simulink model "CxTh_Suff_Neurosci_2004"  (Simulink 6.2)
settings: Solver=ode5  SolverMode=SingleTasking  StartTime=0.0  StopTime=30  FixedStep=0.001  MaxStep=0.01  RelTol=1e-3
libraries: simulink x18
settings Model: LastModifiedBy=Piotr Suffczynski  ExtModeAutoUpdateStatusClock=off
settings SolverCC: InitialStep=0.001
settings DataIOCC: SaveOutput=off  SaveTime=off  SignalLoggingName=sigsOut
settings OptimizationCC: BooleanDataType=off
settings DebuggingCC: CheckMatrixSingularityMsg=warning
settings HardwareCC: TargetUnknown=on
settings GRTTargetCC: ModelReferenceCompliant=off  MatFileLogging=off

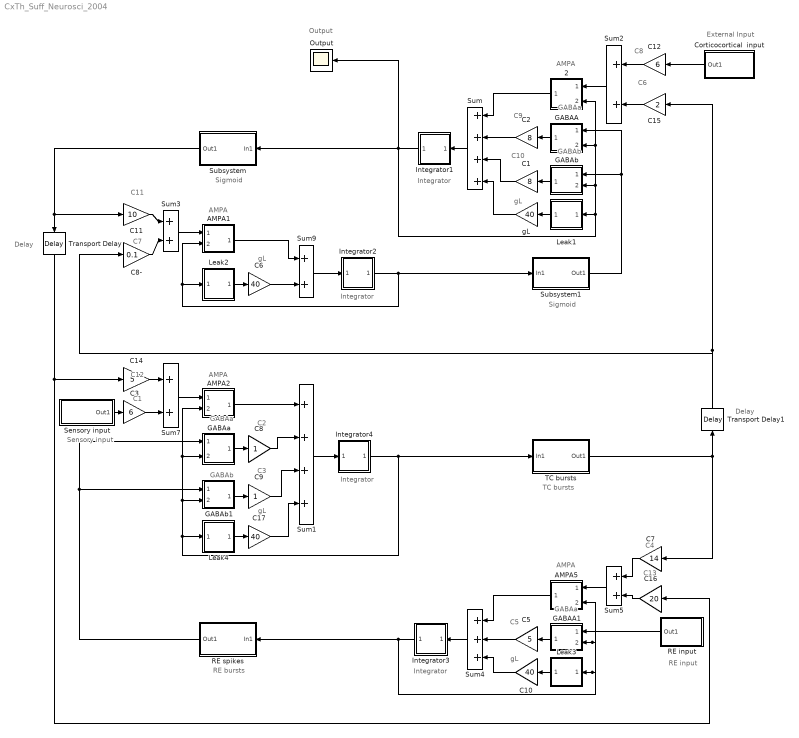
== system CxTh_Suff_Neurosci_2004 ==
  note: Integrator
  note: GABAa
  note: GABAb
  note: AMPA
  note: Sigmoid
  note: AMPA
  note: GABAb
  note: GABAa
  note: AMPA
  note: GABAa
  note: AMPA
  note: External Input
  note: Delay
  note: Delay
  note: Sensory input
  note: RE input
  note: Integrator
  note: Integrator
  note: Integrator
  note: TC bursts
  note: RE bursts
  note: C1
  note: C2
  note: C3
  note: gL
  note: gL
  note: C4
  note: C5
  note: gL
  note: C6
  note: C7
  note: C8
  note: C9
  note: C10
  note: gL
  note: C11
  note: C12
  note: C13
  note: Sigmoid
  note: Output
  2 : Subsystem  Orientation=left
      mask Display: plot([0 5 10 15 20 30 40 60 80 100 150 350], [0  0.3 0.8 1 0.75 0.42 0.22 0.1 0.03 0.01 0 0])
  AMPA1 : Subsystem
      mask Display: plot([0 5 10 15 20 30 40 60 80 100 150 350], [0  0.3 0.8 1 0.75 0.42 0.22 0.1 0.03 0.01 0 0])
  AMPA2 : Subsystem
      mask Display: plot([0 5 10 15 20 30 40 60 80 100 150 350], [0  0.3 0.8 1 0.75 0.42 0.22 0.1 0.03 0.01 0 0])
  AMPA5 : Subsystem  Orientation=left
      mask Display: plot([0 5 10 15 20 30 40 60 80 100 150 350], [0  0.3 0.8 1 0.75 0.42 0.22 0.1 0.03 0.01 0 0])
  C1 : Gain  Orientation=left  Gain=8  SaturateOnIntegerOverflow=on
  C10 : Gain  Orientation=left  Gain=40  SaturateOnIntegerOverflow=on
  C11 : Gain  Gain=10  SaturateOnIntegerOverflow=on
  C12 : Gain  Orientation=left  Gain=6  SaturateOnIntegerOverflow=on
  C14 : Gain  Gain=5  SaturateOnIntegerOverflow=on
  C15 : Gain  Orientation=left  Gain=2  SaturateOnIntegerOverflow=on
  C16 : Gain  Orientation=left  Gain=20  SaturateOnIntegerOverflow=on
  C17 : Gain  Gain=40  SaturateOnIntegerOverflow=on
  C2 : Gain  Orientation=left  Gain=8  SaturateOnIntegerOverflow=on
  C3 : Gain  Gain=6  SaturateOnIntegerOverflow=on
  C5 : Gain  Orientation=left  Gain=5  SaturateOnIntegerOverflow=on
  C6 : Gain  Gain=40  SaturateOnIntegerOverflow=on
  C7 : Gain  Orientation=left  Gain=14  SaturateOnIntegerOverflow=on
  C8 : Gain  SaturateOnIntegerOverflow=on
  C8- : Gain  Gain=0.1
  C9 : Gain  SaturateOnIntegerOverflow=on
  Corticocortical  input : Subsystem  Orientation=left
      mask Display: plot([1 2 3 4 5 6 7 8 9 10 11 12],[0 3 -2 5 1 -2 6 -4 -1 2 -1 0])
  GABAA : Subsystem  Orientation=left
      mask Display: plot([10 15 20 30 40 60 80 100 150 350], [0  0.5 1 0.75 0.5 0.3 0.2 0.1 0.01 0 ])
  GABAA1 : Subsystem  Orientation=left
      mask Display: plot([10 15 20 30 40 60 80 100 150 350], [0  0.5 1 0.75 0.5 0.3 0.2 0.1 0.01 0 ])
  GABAa : Subsystem
      mask Display: plot([10 15 20 30 40 60 80 100 150 350], [0  0.5 1 0.75 0.5 0.3 0.2 0.1 0.01 0 ])
  GABAb : Subsystem  Orientation=left
      mask Display:
      | plot([0 10 20 30 40 50 60 70 80 90 100 125 150 200 250 300],
      | [0 3 7 8  7.5 6.5 5.5 4.5 3.5 2.8 2.2 1.2 0.6 0.2 0.1 0])
  GABAb1 : Subsystem
      mask Display:
      | plot([0 10 20 30 40 50 60 70 80 90 100 125 150 200 250 300],
      | [0 3 7 8  7.5 6.5 5.5 4.5 3.5 2.8 2.2 1.2 0.6 0.2 0.1 0])
  Integrator1 : Subsystem  Orientation=left
      mask Display:
      | plot([ 1 2 3 4 5 6 7 8 9 10 ] - 2,
      |  [0 0 0.5  2  4 6 8  9.5 10 10], -4, 0, 15, 10 )
      | disp('    dt')
  Integrator2 : Subsystem
      mask Display:
      | plot([ 1 2 3 4 5 6 7 8 9 10 ] - 2,
      |  [0 0 0.5  2  4 6 8  9.5 10 10], -4, 0, 15, 10 )
      | disp('    dt')
  Integrator3 : Subsystem  Orientation=left
      mask Display:
      | plot([ 1 2 3 4 5 6 7 8 9 10 ] - 2,
      |  [0 0 0.5  2  4 6 8  9.5 10 10], -4, 0, 15, 10 )
      | disp('    dt')
  Integrator4 : Subsystem
      mask Display:
      | plot([ 1 2 3 4 5 6 7 8 9 10 ] - 2,
      |  [0 0 0.5  2  4 6 8  9.5 10 10], -4, 0, 15, 10 )
      | disp('    dt')
  Leak1 : Subsystem  Orientation=left
      mask Display: disp('Leak')
  Leak2 : Subsystem
      mask Display: disp('Leak')
  Leak3 : Subsystem  Orientation=left
      mask Display: disp('Leak')
  Leak4 : Subsystem
      mask Display: disp('Leak')
  Output : Scope
      settings: TickLabels=on  TimeRange=5  YMin=-1.5  YMax=2  SaveName=V_Cx  DataFormat=Array  MaxDataPoints=100000
  RE input : Subsystem  Orientation=left
      mask Display: plot([0 0 0 20 30 40],[ 0 1 0.3 0.3 0.3 0.3])
  RE spikes : Subsystem  Orientation=left
      mask Display:
      | plot([0 10 20 30 40 50 60 70 80 90 100 110 120 130 140 150 160],
      | [0 0 1 1.9  3.5 5 5.25 5.5 4.5 3.8 3.3 2.2 1.2 0.6 0.2 0.1 0])
      | 
      | plot([50 50], [5 20],  [54 54], [5.1 20], [58 58], [5.2 20], [62 62], [5.3 20], [66 66], [5.4 20],   [70 70], [5.5 20] )
  Sensory input : Subsystem
      mask Display: plot([1 2 3 4 5 6 7 8 9 10 11 12],[0 3 -7 3 -1 2 5 -6 4 2 -4 0])
  Subsystem : Subsystem  Orientation=left
      mask Display:
      | plot(-[0 1 2 3 4 5 6 7 8 9 10 11],
      |  [0 0 0 0.5  2  4 6 8  9.5 10 10 10], 0.1, 0, -10.1, 10 )
  Subsystem1 : Subsystem
      mask Display:
      | plot([0 1 2 3 4 5 6 7 8 9 10 11],
      |  [0 0 0 0.5  2  4 6 8  9.5 10 10 10], -0.1, 0, 10.1, 10 )
  Sum : Sum  Orientation=left  Inputs=++++  SaturateOnIntegerOverflow=on  InputSameDT=on
  Sum1 : Sum  Inputs=4  SaturateOnIntegerOverflow=on  InputSameDT=on
  Sum2 : Sum  Orientation=left  SaturateOnIntegerOverflow=on  InputSameDT=on
  Sum3 : Sum  SaturateOnIntegerOverflow=on  InputSameDT=on
  Sum4 : Sum  Orientation=left  Inputs=+++  SaturateOnIntegerOverflow=on  InputSameDT=on
  Sum5 : Sum  Orientation=left  SaturateOnIntegerOverflow=on  InputSameDT=on
  Sum7 : Sum  SaturateOnIntegerOverflow=on  InputSameDT=on
  Sum9 : Sum  SaturateOnIntegerOverflow=on  InputSameDT=on
  TC bursts : Subsystem
      mask Display:
      | plot([0 10 20 30 40 50 60 70 80 90 100 110 120 130 140 150 160],
      | [0 0 1 1.9  3.5 5 5.25 5.5 4.5 3.8 3.3 2.2 1.2 0.6 0.2 0.1 0])
      | 
      | plot([50 50], [5 20],  [54 54], [5.1 20], [58 58], [5.2 20], [62 62], [5.3 20], [66 66], [5.4 20],   [70 70], [5.5 20] )
  Transport Delay : TransportDelay  Orientation=down  DelayTime=0.008
  Transport Delay1 : TransportDelay  Orientation=up  DelayTime=0.008
  gL : Gain  Orientation=left  Gain=40  SaturateOnIntegerOverflow=on
  wires:
  C8-/1 -> Sum3/2
  C11/1 -> Sum3/1
  Sum3/1 -> AMPA1/1(In1)
  GABAA/1(Out1) -> C2/1
  GABAb/1(Out1) -> C1/1
  Sum/1 -> Integrator1/1(In1)
  Integrator2/1(Out1) -> AMPA1/2(In2), Leak2/1(In2), Subsystem1/1(In1)
  Subsystem1/1(Out1) -> GABAA/1(In1), GABAb/1(In1)
  Sum2/1 -> 2/1(In1)
  C15/1 -> Sum2/2
  RE spikes/1(Out1) -> GABAa/1(In1), GABAb1/1(In1)
  RE input/1(Out1) -> GABAA1/1(In1)
  Sum1/1 -> Integrator4/1(In1)
  TC bursts/1(Out1) -> Transport Delay1/1, C7/1
  GABAb1/1(Out1) -> C9/1
  GABAa/1(Out1) -> C8/1
  AMPA5/1(Out1) -> Sum4/1
  Sum4/1 -> Integrator3/1(In1)
  C7/1 -> Sum5/1
  AMPA2/1(Out1) -> Sum1/1
  Sum7/1 -> AMPA2/1(In1)
  C14/1 -> Sum7/1
  Leak4/1(Out1) -> C17/1
  C17/1 -> Sum1/4
  Transport Delay/1 -> C16/1, C14/1
  Transport Delay1/1 -> C15/1, C8-/1
  C2/1 -> Sum/2
  C1/1 -> Sum/3
  Subsystem/1(Out1) -> Transport Delay/1, C11/1
  C8/1 -> Sum1/2
  C9/1 -> Sum1/3
  Leak1/1(Out1) -> gL/1
  gL/1 -> Sum/4
  Leak2/1(Out1) -> C6/1
  C6/1 -> Sum9/2
  Sum9/1 -> Integrator2/1(In1)
  Leak3/1(Out1) -> C10/1
  C10/1 -> Sum4/3
  C16/1 -> Sum5/2
  Integrator4/1(Out1) -> GABAa/2(In2), AMPA2/2(In2), GABAb1/2(In2), Leak4/1(In2), TC bursts/1(In1)
  Integrator3/1(Out1) -> RE spikes/1(In1), AMPA5/2(In2), GABAA1/2(In2), Leak3/1(In2)
  Sum5/1 -> AMPA5/1(In1)
  2/1(Out1) -> Sum/1
  AMPA1/1(Out1) -> Sum9/1
  C5/1 -> Sum4/2
  GABAA1/1(Out1) -> C5/1
  Integrator1/1(Out1) -> Subsystem/1(In1), Leak1/1(In2), GABAb/2(In2), 2/2(In2), GABAA/2(In2), Output/1
  C3/1 -> Sum7/2
  Sensory input/1(Out1) -> C3/1
  Corticocortical  input/1(Out1) -> C12/1
  C12/1 -> Sum2/1

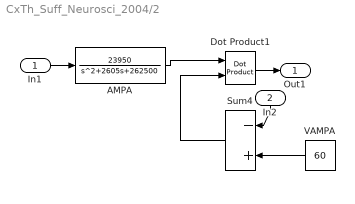
== system CxTh_Suff_Neurosci_2004/2 ==
  In1 : Inport  Port=1  LatchInput=off
  In2 : Inport  Orientation=down  Port=2  LatchInput=off
  AMPA : TransferFcn  Numerator=[23950]  Denominator="[1  2605 262500]"
  Dot Product1 : simulink/Math Operations/Dot Product  InputSameDT=on  OutDataType=sfix(16)  OutScaling=2^-10  DoSatur=off
  Sum4 : Sum  Orientation=left  Inputs=-+  SaturateOnIntegerOverflow=on  InputSameDT=on
  VAMPA : Constant  Orientation=left  Value=60
  Out1 : Outport
  wires:
  Dot Product1/1 -> Out1/1
  In1/1 -> AMPA/1
  In2/1 -> Sum4/1
  Sum4/1 -> Dot Product1/2
  VAMPA/1 -> Sum4/2
  AMPA/1 -> Dot Product1/1

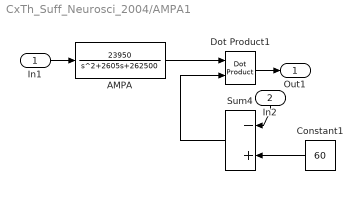
== system CxTh_Suff_Neurosci_2004/AMPA1 ==
  In1 : Inport  Port=1  LatchInput=off
  In2 : Inport  Orientation=down  Port=2  LatchInput=off
  AMPA : TransferFcn  Numerator=[23950]  Denominator="[1  2605 262500]"
  Constant1 : Constant  Orientation=left  Value=60
  Dot Product1 : simulink/Math Operations/Dot Product  InputSameDT=on  OutDataType=sfix(16)  OutScaling=2^-10  DoSatur=off
  Sum4 : Sum  Orientation=left  Inputs=-+  SaturateOnIntegerOverflow=on  InputSameDT=on
  Out1 : Outport
  wires:
  AMPA/1 -> Dot Product1/1
  Constant1/1 -> Sum4/2
  Sum4/1 -> Dot Product1/2
  In2/1 -> Sum4/1
  In1/1 -> AMPA/1
  Dot Product1/1 -> Out1/1

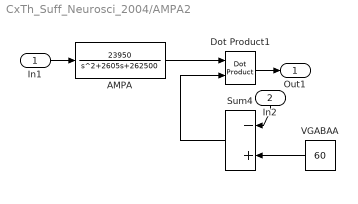
== system CxTh_Suff_Neurosci_2004/AMPA2 ==
  In1 : Inport  Port=1  LatchInput=off
  In2 : Inport  Orientation=down  Port=2  LatchInput=off
  AMPA : TransferFcn  Numerator=[23950]  Denominator="[1  2605 262500]"
  Dot Product1 : simulink/Math Operations/Dot Product  InputSameDT=on  OutDataType=sfix(16)  OutScaling=2^-10  DoSatur=off
  Sum4 : Sum  Orientation=left  Inputs=-+  SaturateOnIntegerOverflow=on  InputSameDT=on
  VGABAA : Constant  Orientation=left  Value=60
  Out1 : Outport
  wires:
  Dot Product1/1 -> Out1/1
  In1/1 -> AMPA/1
  In2/1 -> Sum4/1
  Sum4/1 -> Dot Product1/2
  VGABAA/1 -> Sum4/2
  AMPA/1 -> Dot Product1/1

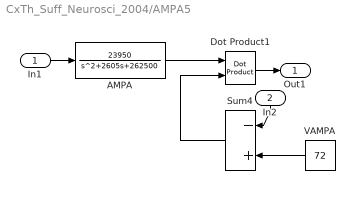
== system CxTh_Suff_Neurosci_2004/AMPA5 ==
  In1 : Inport  Port=1  LatchInput=off
  In2 : Inport  Orientation=down  Port=2  LatchInput=off
  AMPA : TransferFcn  Numerator=[23950]  Denominator="[1  2605 262500]"
  Dot Product1 : simulink/Math Operations/Dot Product  InputSameDT=on  OutDataType=sfix(16)  OutScaling=2^-10  DoSatur=off
  Sum4 : Sum  Orientation=left  Inputs=-+  SaturateOnIntegerOverflow=on  InputSameDT=on
  VAMPA : Constant  Orientation=left  Value=72
  Out1 : Outport
  wires:
  AMPA/1 -> Dot Product1/1
  VAMPA/1 -> Sum4/2
  Sum4/1 -> Dot Product1/2
  In2/1 -> Sum4/1
  In1/1 -> AMPA/1
  Dot Product1/1 -> Out1/1

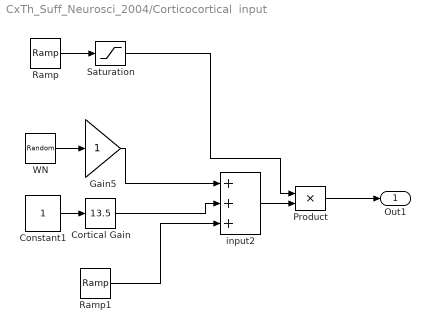
== system CxTh_Suff_Neurosci_2004/Corticocortical  input ==
  Constant1 : Constant
  Cortical Gain : simulink/Math Operations/Slider Gain  low=0  gain=13.5  high=200
  Gain5 : Gain  SaturateOnIntegerOverflow=on
  Product : Product  SaturateOnIntegerOverflow=on  InputSameDT=on
  Ramp : simulink/Sources/Ramp  slope=0.2  start=0  X0=0
  Ramp1 : simulink/Sources/Ramp  slope=0  start=0  X0=0
  Saturation : Saturate  UpperLimit=1  LowerLimit=0
  WN : RandomNumber  SampleTime=0.001
  input2 : Sum  Inputs=+++  SaturateOnIntegerOverflow=on  InputSameDT=on
  Out1 : Outport  InitialOutput=0
  wires:
  Cortical Gain/1 -> input2/2
  WN/1 -> Gain5/1
  Gain5/1 -> input2/1
  Constant1/1 -> Cortical Gain/1
  Saturation/1 -> Product/1
  Ramp/1 -> Saturation/1
  input2/1 -> Product/2
  Product/1 -> Out1/1
  Ramp1/1 -> input2/3

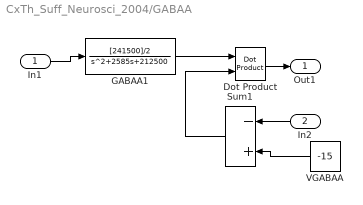
== system CxTh_Suff_Neurosci_2004/GABAA ==
  In1 : Inport  Port=1  LatchInput=off
  In2 : Inport  Orientation=left  Port=2  LatchInput=off
  Dot Product : simulink/Math Operations/Dot Product  InputSameDT=on  OutDataType=sfix(16)  OutScaling=2^-10  DoSatur=off
  GABAA1 : TransferFcn  Numerator=[241500]/2  Denominator="[1  2585 212500]"
  Sum1 : Sum  Orientation=left  Inputs=-+  SaturateOnIntegerOverflow=on  InputSameDT=on
  VGABAA : Constant  Orientation=left  Value=-15
  Out1 : Outport
  wires:
  GABAA1/1 -> Dot Product/1
  VGABAA/1 -> Sum1/2
  Sum1/1 -> Dot Product/2
  In1/1 -> GABAA1/1
  In2/1 -> Sum1/1
  Dot Product/1 -> Out1/1

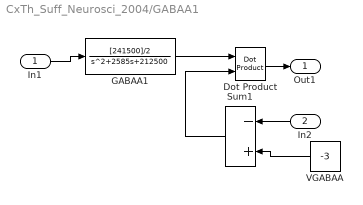
== system CxTh_Suff_Neurosci_2004/GABAA1 ==
  In1 : Inport  Port=1  LatchInput=off
  In2 : Inport  Orientation=left  Port=2  LatchInput=off
  Dot Product : simulink/Math Operations/Dot Product  InputSameDT=on  OutDataType=sfix(16)  OutScaling=2^-10  DoSatur=off
  GABAA1 : TransferFcn  Numerator=[241500]/2  Denominator="[1  2585 212500]"
  Sum1 : Sum  Orientation=left  Inputs=-+  SaturateOnIntegerOverflow=on  InputSameDT=on
  VGABAA : Constant  Orientation=left  Value=-3
  Out1 : Outport
  wires:
  Dot Product/1 -> Out1/1
  In2/1 -> Sum1/1
  In1/1 -> GABAA1/1
  Sum1/1 -> Dot Product/2
  VGABAA/1 -> Sum1/2
  GABAA1/1 -> Dot Product/1

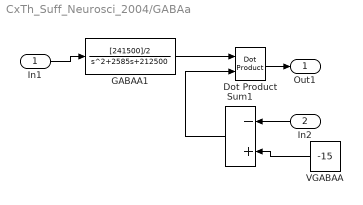
== system CxTh_Suff_Neurosci_2004/GABAa ==
  In1 : Inport  Port=1  LatchInput=off
  In2 : Inport  Orientation=left  Port=2  LatchInput=off
  Dot Product : simulink/Math Operations/Dot Product  InputSameDT=on  OutDataType=sfix(16)  OutScaling=2^-10  DoSatur=off
  GABAA1 : TransferFcn  Numerator=[241500]/2  Denominator="[1  2585 212500]"
  Sum1 : Sum  Orientation=left  Inputs=-+  SaturateOnIntegerOverflow=on  InputSameDT=on
  VGABAA : Constant  Orientation=left  Value=-15
  Out1 : Outport
  wires:
  GABAA1/1 -> Dot Product/1
  VGABAA/1 -> Sum1/2
  Sum1/1 -> Dot Product/2
  In1/1 -> GABAA1/1
  In2/1 -> Sum1/1
  Dot Product/1 -> Out1/1

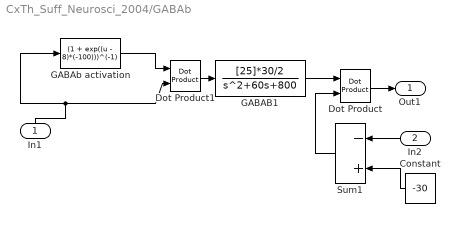
== system CxTh_Suff_Neurosci_2004/GABAb ==
  In1 : Inport  Orientation=up  Port=1  LatchInput=off
  In2 : Inport  Orientation=left  Port=2  LatchInput=off
  Constant : Constant  Orientation=left  Value=-30
  Dot Product : simulink/Math Operations/Dot Product  InputSameDT=on  OutDataType=sfix(16)  OutScaling=2^-10  DoSatur=off
  Dot Product1 : simulink/Math Operations/Dot Product  InputSameDT=on  OutDataType=sfix(16)  OutScaling=2^-10  DoSatur=off
  GABAB1 : TransferFcn  Numerator=[25]*30/2  Denominator="[1  60 800]"
  GABAb activation : Fcn  Expr=(1 + exp((u - 8)*(-100)))^(-1)
  Sum1 : Sum  Orientation=left  Inputs=-+  SaturateOnIntegerOverflow=on  InputSameDT=on
  Out1 : Outport
  wires:
  GABAB1/1 -> Dot Product/1
  Constant/1 -> Sum1/2
  Sum1/1 -> Dot Product/2
  Dot Product1/1 -> GABAB1/1
  In1/1 -> Dot Product1/2, GABAb activation/1
  In2/1 -> Sum1/1
  Dot Product/1 -> Out1/1
  GABAb activation/1 -> Dot Product1/1

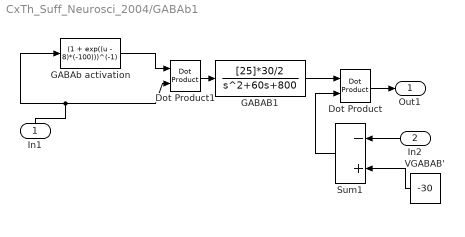
== system CxTh_Suff_Neurosci_2004/GABAb1 ==
  In1 : Inport  Orientation=up  Port=1  LatchInput=off
  In2 : Inport  Orientation=left  Port=2  LatchInput=off
  Dot Product : simulink/Math Operations/Dot Product  InputSameDT=on  OutDataType=sfix(16)  OutScaling=2^-10  DoSatur=off
  Dot Product1 : simulink/Math Operations/Dot Product  InputSameDT=on  OutDataType=sfix(16)  OutScaling=2^-10  DoSatur=off
  GABAB1 : TransferFcn  Numerator=[25]*30/2  Denominator="[1  60 800]"
  GABAb activation : Fcn  Expr=(1 + exp((u - 8)*(-100)))^(-1)
  Sum1 : Sum  Orientation=left  Inputs=-+  SaturateOnIntegerOverflow=on  InputSameDT=on
  VGABAB' : Constant  Orientation=left  Value=-30
  Out1 : Outport
  wires:
  GABAb activation/1 -> Dot Product1/1
  Dot Product/1 -> Out1/1
  In2/1 -> Sum1/1
  In1/1 -> GABAb activation/1, Dot Product1/2
  Dot Product1/1 -> GABAB1/1
  Sum1/1 -> Dot Product/2
  VGABAB'/1 -> Sum1/2
  GABAB1/1 -> Dot Product/1

== system CxTh_Suff_Neurosci_2004/Integrator1 ==
  In1 : Inport  Port=1  LatchInput=off
  Integrator2 : Integrator
  Out1 : Outport
  wires:
  In1/1 -> Integrator2/1
  Integrator2/1 -> Out1/1

== system CxTh_Suff_Neurosci_2004/Integrator2 ==
  In1 : Inport  Port=1  LatchInput=off
  Integrator2 : Integrator
  Out1 : Outport
  wires:
  Integrator2/1 -> Out1/1
  In1/1 -> Integrator2/1

== system CxTh_Suff_Neurosci_2004/Integrator3 ==
  In1 : Inport  Port=1  LatchInput=off
  Integrator2 : Integrator
  Out1 : Outport
  wires:
  Integrator2/1 -> Out1/1
  In1/1 -> Integrator2/1

== system CxTh_Suff_Neurosci_2004/Integrator4 ==
  In1 : Inport  Port=1  LatchInput=off
  Integrator2 : Integrator
  Out1 : Outport
  wires:
  In1/1 -> Integrator2/1
  Integrator2/1 -> Out1/1

== system CxTh_Suff_Neurosci_2004/Leak1 ==
  In2 : Inport  Orientation=left  Port=1  LatchInput=off
  Sum1 : Sum  Orientation=left  Inputs=-+  SaturateOnIntegerOverflow=on  InputSameDT=on
  Vleak : Constant  Orientation=left  Value=0
  Out1 : Outport
  wires:
  Vleak/1 -> Sum1/2
  In2/1 -> Sum1/1
  Sum1/1 -> Out1/1

== system CxTh_Suff_Neurosci_2004/Leak2 ==
  In2 : Inport  Orientation=left  Port=1  LatchInput=off
  Sum1 : Sum  Orientation=left  Inputs=-+  SaturateOnIntegerOverflow=on  InputSameDT=on
  Vleak : Constant  Orientation=left  Value=0
  Out1 : Outport
  wires:
  Sum1/1 -> Out1/1
  In2/1 -> Sum1/1
  Vleak/1 -> Sum1/2

== system CxTh_Suff_Neurosci_2004/Leak3 ==
  In2 : Inport  Orientation=left  Port=1  LatchInput=off
  Sum1 : Sum  Orientation=left  Inputs=-+  SaturateOnIntegerOverflow=on  InputSameDT=on
  Vleak : Constant  Orientation=left  Value=0
  Out1 : Outport
  wires:
  Vleak/1 -> Sum1/2
  In2/1 -> Sum1/1
  Sum1/1 -> Out1/1

== system CxTh_Suff_Neurosci_2004/Leak4 ==
  In2 : Inport  Orientation=left  Port=1  LatchInput=off
  Sum1 : Sum  Orientation=left  Inputs=-+  SaturateOnIntegerOverflow=on  InputSameDT=on
  Vleak : Constant  Orientation=left  Value=0
  Out1 : Outport
  wires:
  Vleak/1 -> Sum1/2
  In2/1 -> Sum1/1
  Sum1/1 -> Out1/1

== system CxTh_Suff_Neurosci_2004/RE input ==
  Constant2 : Constant  Orientation=left  Value=12
  Out1 : Outport  Orientation=left
  wires:
  Constant2/1 -> Out1/1

== system CxTh_Suff_Neurosci_2004/RE spikes ==
  In1 : Inport  Orientation=left  Port=1  LatchInput=off
  C_RE : Gain  Orientation=left  Gain=800  SaturateOnIntegerOverflow=on
  LTS_RE1 : Subsystem  Orientation=left
  Out1 : Outport  Orientation=left
  wires:
  LTS_RE1/1(Out1) -> C_RE/1
  In1/1 -> LTS_RE1/1(In1)
  C_RE/1 -> Out1/1

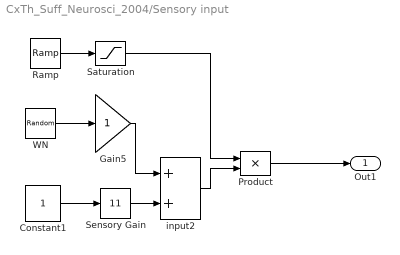
== system CxTh_Suff_Neurosci_2004/Sensory input ==
  Constant1 : Constant
  Gain5 : Gain  SaturateOnIntegerOverflow=on
  Product : Product  SaturateOnIntegerOverflow=on  InputSameDT=on
  Ramp : simulink/Sources/Ramp  slope=0.2  start=0  X0=0
  Saturation : Saturate  UpperLimit=1  LowerLimit=0
  Sensory Gain : simulink/Math Operations/Slider Gain  low=0  gain=11  high=100
  WN : RandomNumber  Seed=2  SampleTime=0.001
  input2 : Sum  SaturateOnIntegerOverflow=on  InputSameDT=on
  Out1 : Outport  InitialOutput=0
  wires:
  Saturation/1 -> Product/1
  Ramp/1 -> Saturation/1
  Product/1 -> Out1/1
  Sensory Gain/1 -> input2/2
  WN/1 -> Gain5/1
  Gain5/1 -> input2/1
  input2/1 -> Product/2
  Constant1/1 -> Sensory Gain/1

== system CxTh_Suff_Neurosci_2004/Subsystem ==
  In1 : Inport  Orientation=left  Port=1  LatchInput=off
  Fcn : Fcn  Orientation=left  Expr=50*(1 + exp((u - 7)/-2))^(-1)
  Out1 : Outport  Orientation=left
  wires:
  In1/1 -> Fcn/1
  Fcn/1 -> Out1/1

== system CxTh_Suff_Neurosci_2004/Subsystem1 ==
  In1 : Inport  Port=1  LatchInput=off
  Fcn1 : Fcn  Expr=50*(1 + exp((u(1) - 7)/(-2)))^(-1)
  Out1 : Outport
  wires:
  In1/1 -> Fcn1/1
  Fcn1/1 -> Out1/1

== system CxTh_Suff_Neurosci_2004/TC bursts ==
  In1 : Inport  Port=1  LatchInput=off
  C_TC : Gain  Gain=800  SaturateOnIntegerOverflow=on
  LTS_TC1 : Subsystem
  Out1 : Outport
  wires:
  LTS_TC1/1(Out1) -> C_TC/1
  In1/1 -> LTS_TC1/1(In1)
  C_TC/1 -> Out1/1

== system CxTh_Suff_Neurosci_2004/RE spikes/LTS_RE1 ==
  In1 : Inport  Port=1  LatchInput=off
  Dot Product : simulink/Math Operations/Dot Product  InputSameDT=on  OutDataType=sfix(16)  OutScaling=2^-10  DoSatur=off
  GABAa1 : TransferFcn  Numerator=[5200]  Denominator=[1 170 5200]
  IT activation : Fcn  Expr=(1 + exp((u - 16)/(-2)))^(-1)
  IT inactivation : Fcn  Expr=(1 + exp((u + 6)/6))^(-1)
  Out1 : Outport
  wires:
  GABAa1/1 -> Dot Product/2
  IT inactivation/1 -> GABAa1/1
  IT activation/1 -> Dot Product/1
  In1/1 -> IT activation/1, IT inactivation/1
  Dot Product/1 -> Out1/1

== system CxTh_Suff_Neurosci_2004/TC bursts/LTS_TC1 ==
  In1 : Inport  Port=1  LatchInput=off
  Dot Product : simulink/Math Operations/Dot Product  InputSameDT=on  OutDataType=sfix(16)  OutScaling=2^-10  DoSatur=off
  GABAa1 : TransferFcn  Numerator=[5200]  Denominator=[1 170 5200]
  IT activation : Fcn  Expr=(1 + exp((u - 6)/(-2)))^(-1)
  IT inactivation : Fcn  Expr=(1 + exp((u + 16)/6))^(-1)
  Out1 : Outport
  wires:
  IT inactivation/1 -> GABAa1/1
  GABAa1/1 -> Dot Product/2
  Dot Product/1 -> Out1/1
  In1/1 -> IT inactivation/1, IT activation/1
  IT activation/1 -> Dot Product/1
